simulink model "Q5"  (R2020b)
settings: Solver=VariableStepAuto  StartTime=0.0  StopTime=10.0  RelTol=1e-3
settings Model: Creator=Javad  LastModifiedBy=Javad
settings SolverCC: ZeroCrossAlgorithm=Adaptive
settings DebuggingCC: IgnoredZcDiagnostic=none

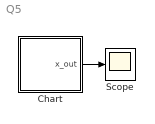
== system Q5 ==
  Chart : Stateflow chart  TreatAsAtomicUnit=on
  Scope : Scope
  wires:
  Chart/1(x_out) -> Scope/1

== stateflow chart Q5/Chart ==
  settings: updateMethod=CONTINUOUS
  state off
    du:
    x_dot=-x;
    x_out=x;
  state on
    du:
    x_dot=-x+100;
    x_out=x;
  (default) -> off : {x=50;}
  off -> on : [x<69]{x=x;}
  on -> off : [x>71]{x=x;}
  data: x_out output; x local
  data x settings: updateMethod=SF_CONTINUOUS_TIME_DATA
